simulink model "ADC_final_simulation"  (R2021a)
settings: Solver=ode4  StartTime=0.0  StopTime=50  FixedStep=0.01  RelTol=1e-3
libraries: mobileRoboticsLib x2, simulink x2, dspinverses x2, dsppolyfun x2
settings Model: Creator=rmml  LastModifiedBy=TigerWUU
settings SolverCC: ZeroCrossAlgorithm=Adaptive  AlgebraicLoopSolver=TrustRegion
settings DebuggingCC: IgnoredZcDiagnostic=none  SFMachineParentedDataDiag=warning

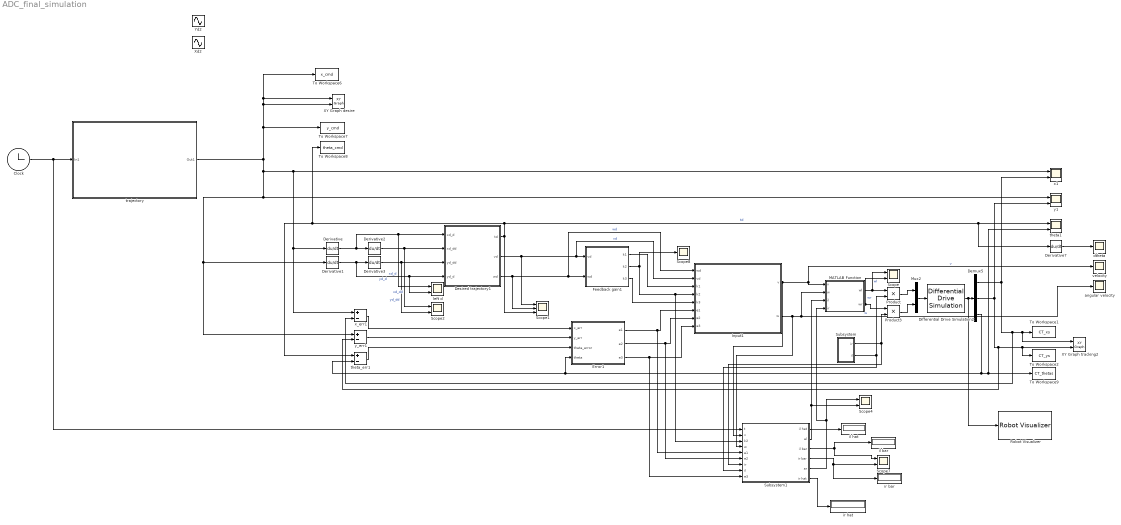
== system ADC_final_simulation ==
  Clock : Clock
  Demux5 : Demux  Outputs=3
  Derivative{,1..3,7} (5 alike) : Derivative  CoefficientInTFapproximation=0
  Desired trajectory1 : MATLAB Function  TreatAsAtomicUnit=on
  Differential Drive Simulation2 : mobileRoboticsLib/Kinematic Models/Differential Drive/Differential Drive Simulation  wheelRadius=0.075  wheelBase=0.3  initX=-0.2  initY=-0.2  initAngle=3*pi/4  Ts=0.01
      settings: SourceProductName=Mobile Robotics Simulation Toolbox
  Error1 : MATLAB Function  TreatAsAtomicUnit=on
  Feedback gain1 : MATLAB Function  TreatAsAtomicUnit=on
  Input1 : MATLAB Function  TreatAsAtomicUnit=on
  MATLAB Function : MATLAB Function  TreatAsAtomicUnit=on
  Mux2 : Mux  Inputs=2
  Product : Product
  Product3 : Product
  Robot Visualizer : mobileRoboticsLib/Environments/Robot Visualizer  robotRadius=0  showTrajectory=on  hasWaypoints=off  hasLidar=off  sensorOffset=[ 0, 0 ]  scanAngles=[ -pi/4, 0, pi/4 ]  hasObjDetector=off  objDetectorOffset=[ 0, 0 ]  objDetectorAngle=0  objDetectorFOV=pi/4  objDetectorMaxRange=5  objectColors=[ 1, 0, 0; 0, 1, 0; 0, 0, 1 ]  objectMarkers='s'
  Scope{,2,4,7} (4 alike) : Scope  NumInputPorts=2
  Scope1 : Scope  NumInputPorts=3
  Scope8 : Scope
  Subsystem : Subsystem
  Subsystem1 : Subsystem
  To Workspace1 : ToWorkspace  VariableName=CT_xs  SampleTime=-1
      settings: Save2DSignal=2-D array (concatenate along first dimension)
  To Workspace2 : ToWorkspace  VariableName=CT_ys  SampleTime=-1
      settings: Save2DSignal=2-D array (concatenate along first dimension)
  To Workspace6 : ToWorkspace  VariableName=x_cmd  SampleTime=-1
      settings: Save2DSignal=2-D array (concatenate along first dimension)
  To Workspace7 : ToWorkspace  VariableName=y_cmd  SampleTime=-1
      settings: Save2DSignal=2-D array (concatenate along first dimension)
  To Workspace8 : ToWorkspace  VariableName=theta_cmd  SampleTime=-1
      settings: Save2DSignal=2-D array (concatenate along first dimension)
  To Workspace9 : ToWorkspace  VariableName=CT_thetas  SampleTime=-1
      settings: Save2DSignal=2-D array (concatenate along first dimension)
  XY Graph desire : simulink/Sinks/XY Graph  xmin=-3  xmax=3  ymin=-3  ymax=3  st=-1
  XY Graph tracking2 : simulink/Sinks/XY Graph  xmin=-3  xmax=3  ymin=-3  ymax=3  st=-1
  Xd2 : Sin  TimeSource=Use external signal  Amplitude=-1.6  SampleTime=0
  Yd2 : Sin  TimeSource=Use external signal  Amplitude=-1.6  Bias=1.6  Phase=pi/2  SampleTime=0
  angular velocity : Scope
  dtheta : Scope
  il bar : Display
  il hat : Display
  ir bar : Display
  ir hat : Display
  left d : Scope  NumInputPorts=2
  theta1 : Scope  NumInputPorts=2
  theta_err1 : Sum  Inputs=+-
  trajectory : Subsystem
  velocity : Scope
  x1 : Scope  NumInputPorts=2
  x_err1 : Sum  Inputs=+-
  y1 : Scope  NumInputPorts=2
  y_err1 : Sum  Inputs=+-
  wires:
  Derivative/1 -> Derivative2/1, left d/1, Desired trajectory1/1(xd_d)  "xd_d"
  Derivative7/1 -> dtheta/1
  Feedback gain1/3(k3) -> Input1/5(k3)
  Derivative1/1 -> Desired trajectory1/4(yd_d), left d/2, Derivative3/1  "yd_d"
  Error1/1(e1) -> Subsystem1/5(e1), Input1/6(e1)
  Input1/1(v) -> Subsystem1/2(v), MATLAB Function/1(v), velocity/1  "v"
  y_err1/1 -> Error1/2(y_err)
  Error1/2(e2) -> Subsystem1/6(e2), Input1/7(e2)
  Desired trajectory1/1(td) -> To Workspace8/1, theta_err1/1, theta1/1, Derivative7/1, Scope1/3  "td"
  x_err1/1 -> Error1/1(x_err)
  Derivative2/1 -> Scope2/1, Desired trajectory1/2(xd_dd)  "xd_dd"
  Input1/2(w) -> Subsystem1/4(w), angular velocity/1, MATLAB Function/2(w)  "w"
  Desired trajectory1/2(vd) -> Scope1/1, Feedback gain1/1(vd), Input1/2(vd)  "vd"
  Feedback gain1/2(k2) -> Scope8/1, Subsystem1/3(k2), Input1/4(k2)
  Desired trajectory1/3(wd) -> Input1/1(wd), Feedback gain1/2(wd), Scope1/2  "wd"
  Clock/1 -> Subsystem1/1(t), trajectory/1(In1)
  Feedback gain1/1(k1) -> Input1/3(k1)
  Derivative3/1 -> Scope2/2, Desired trajectory1/3(yd_dd)  "yd_dd"
  Error1/3(e3) -> Subsystem1/9(e3), Input1/8(e3)
  theta_err1/1 -> Error1/3(theta_error)
  MATLAB Function/1(wl) -> Scope/1, Product/1  "wl"
  MATLAB Function/2(wr) -> Scope/2, Product3/1  "wr"
  Mux2/1 -> Differential Drive Simulation2/1
  Differential Drive Simulation2/1 -> Robot Visualizer/1, Demux5/1
  Demux5/1 -> x_err1/2, XY Graph tracking2/1, To Workspace1/1, x1/2
  Demux5/2 -> y_err1/2, To Workspace2/1, XY Graph tracking2/2, y1/2
  Product/1 -> Mux2/1
  Product3/1 -> Mux2/2
  Demux5/3 -> theta1/2, To Workspace9/1, Error1/4(theta), theta_err1/2
  trajectory/1(Out1) -> x1/1, x_err1/1, Derivative/1, Derivative1/1, y_err1/1, y1/1, To Workspace6/1, XY Graph desire/1, XY Graph desire/2, To Workspace7/1
  Subsystem/1(ir) -> Subsystem1/7(ir), Product3/2
  Subsystem/2(il) -> Subsystem1/8(il), Product/2
  Subsystem1/4(ir bar) -> ir bar/1, Scope7/2
  Subsystem1/3(il bar) -> Scope7/1, il bar/1
  Subsystem1/2(al) -> Scope4/2, MATLAB Function/3(il)
  Subsystem1/5(ar) -> MATLAB Function/4(ir), Scope4/1
  Subsystem1/1(il hat) -> il hat/1
  Subsystem1/6(ir hat) -> ir hat/1

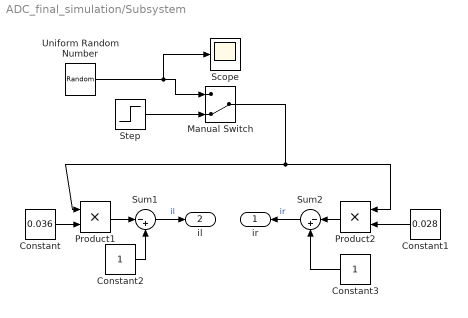
== system ADC_final_simulation/Subsystem ==
  Constant : Constant  Value=0.036
  Constant1 : Constant  Value=0.028
  Constant2 : Constant
  Constant3 : Constant
  Manual Switch : ManualSwitch  CurrentSetting=0
  Product1 : Product
  Product2 : Product
  Scope : Scope
  Step : Step  Time=20  SampleTime=0
  Sum1 : Sum  Inputs=|-+
  Sum2 : Sum  Inputs=|-+
  Uniform Random Number : UniformRandomNumber  SampleTime=0.1
  ir : Outport
  il : Outport  Port=2
  wires:
  Sum1/1 -> il/1  "il"
  Constant3/1 -> Sum2/2
  Product1/1 -> Sum1/1
  Product2/1 -> Sum2/1
  Constant2/1 -> Sum1/2
  Sum2/1 -> ir/1  "ir"
  Constant1/1 -> Product2/2
  Constant/1 -> Product1/2
  Step/1 -> Manual Switch/2
  Uniform Random Number/1 -> Scope/1, Manual Switch/1
  Manual Switch/1 -> Product2/1, Product1/1

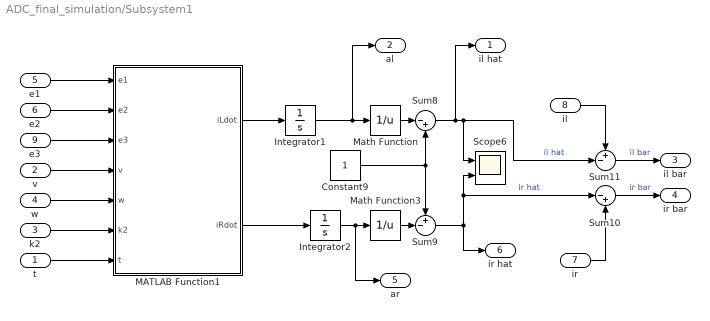
== system ADC_final_simulation/Subsystem1 ==
  t : Inport
  v : Inport  Port=2
  k2 : Inport  Port=3
  w : Inport  Port=4
  e1 : Inport  Port=5
  e2 : Inport  Port=6
  ir : Inport  Port=7
  il : Inport  Port=8
  e3 : Inport  Port=9
  Constant9 : Constant
  Integrator1 : Integrator
  Integrator2 : Integrator
  MATLAB Function1 : MATLAB Function  TreatAsAtomicUnit=on
  Math Function : Math  Operator=reciprocal  SaturateOnIntegerOverflow=on
  Math Function3 : Math  Operator=reciprocal  SaturateOnIntegerOverflow=on
  Scope6 : Scope  NumInputPorts=2
  Sum10 : Sum  Inputs=|-+
  Sum11 : Sum  Inputs=+-|
  Sum8 : Sum  Inputs=|-+
  Sum9 : Sum  Inputs=+-|
  il hat : Outport
  al : Outport  Port=2
  il bar : Outport  Port=3
  ir bar : Outport  Port=4
  ar : Outport  Port=5
  ir hat : Outport  Port=6
  wires:
  e2/1 -> MATLAB Function1/2(e2)
  Math Function/1 -> Sum8/1
  Integrator1/1 -> al/1, Math Function/1
  Integrator2/1 -> ar/1, Math Function3/1
  Constant9/1 -> Sum8/2, Sum9/1
  e3/1 -> MATLAB Function1/3(e3)
  w/1 -> MATLAB Function1/5(w)
  Sum8/1 -> il hat/1, Scope6/1, Sum11/2  "il hat"
  MATLAB Function1/2(iRdot) -> Integrator2/1
  Sum9/1 -> Scope6/2, Sum10/1, ir hat/1  "ir hat"
  Sum10/1 -> ir bar/1  "ir bar"
  t/1 -> MATLAB Function1/7(t)
  MATLAB Function1/1(iLdot) -> Integrator1/1
  Math Function3/1 -> Sum9/2
  Sum11/1 -> il bar/1  "il bar"
  k2/1 -> MATLAB Function1/6(k2)
  v/1 -> MATLAB Function1/4(v)
  e1/1 -> MATLAB Function1/1(e1)
  ir/1 -> Sum10/2
  il/1 -> Sum11/1

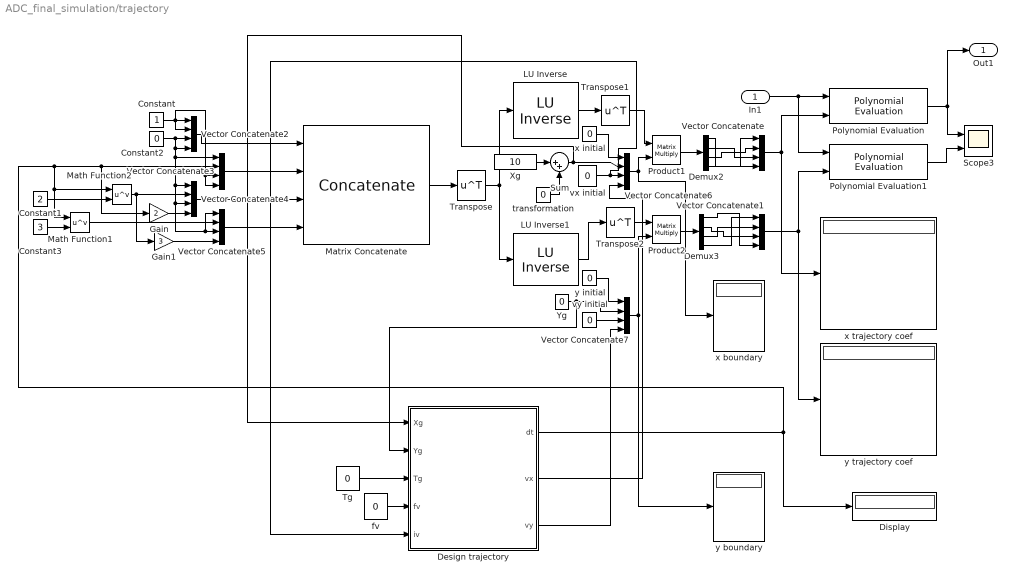
== system ADC_final_simulation/trajectory ==
  In1 : Inport
  " LU Inverse" : dspinverses/ LU Inverse
  " LU Inverse1" : dspinverses/ LU Inverse
  Constant : Constant
  Constant1 : Constant  Value=2
  Constant2 : Constant  Value=0
  Constant3 : Constant  Value=3
  Demux2 : Demux
  Demux3 : Demux
  Design trajectory : MATLAB Function  TreatAsAtomicUnit=on
  Display : Display
  Gain : Gain  Gain=2
  Gain1 : Gain  Gain=3
  Math Function1 : Math  Operator=pow  SaturateOnIntegerOverflow=on
  Math Function2 : Math  Operator=pow  SaturateOnIntegerOverflow=on
  Matrix Concatenate : Concatenate  NumInputs=4  Mode=Multidimensional array  ConcatenateDimension=2
  Polynomial Evaluation : dsppolyfun/Polynomial Evaluation  useConstCoeffs=off  constCoeffs=[5 4 3 2]
      settings: SourceProductBaseCode=DS
  Polynomial Evaluation1 : dsppolyfun/Polynomial Evaluation  useConstCoeffs=off  constCoeffs=[5 4 3 2]
      settings: SourceProductBaseCode=DS
  Product1 : Product  Multiplication=Matrix(*)
  Product2 : Product  Multiplication=Matrix(*)
  Scope3 : Scope  NumInputPorts=2
  Sum : Sum  Inputs=|++
  Tg : Constant  Value=0
  Transpose : Math  Operator=transpose  SaturateOnIntegerOverflow=on
  Transpose1 : Math  Operator=transpose  SaturateOnIntegerOverflow=on
  Transpose2 : Math  Operator=transpose  SaturateOnIntegerOverflow=on
  Vector Concatenate{,1..7} (8 alike) : Concatenate  NumInputs=4
  "Xg " : Constant  Value=10
  Yg : Constant  Value=0
  fv : Constant  Value=0
  transformation : Constant  Value=0
  "vx initial " : Constant  Value=0
  "vy initial " : Constant  Value=0
  "x boundary " : Display
  "x initial " : Constant  Value=0
  x trajectory coef : Display
  "y boundary " : Display
  "y initial " : Constant  Value=0
  y trajectory coef : Display
  Out1 : Outport
  wires:
  Polynomial Evaluation1/1 -> Scope3/2
  Product2/1 -> Demux3/1
  Yg/1 -> Design trajectory/2(Yg), Vector Concatenate7/2
  Math Function2/1 -> Gain1/1, Vector Concatenate4/2
  "vy initial "/1 -> Vector Concatenate7/3
  Tg/1 -> Design trajectory/3(Tg)
  Demux2/2 -> Vector Concatenate/3
  Constant/1 -> Vector Concatenate2/1, Vector Concatenate3/4, Vector Concatenate3/3, Vector Concatenate2/2
  fv/1 -> Design trajectory/4(fv)
  Vector Concatenate3/1 -> Matrix Concatenate/2
  Vector Concatenate5/1 -> Matrix Concatenate/4
  Vector Concatenate6/1 -> "x boundary "/1, Product1/2
  Vector Concatenate7/1 -> Product2/2, "y boundary "/1
  transformation/1 -> Sum/2
  Constant2/1 -> Vector Concatenate5/3, Vector Concatenate5/1, Vector Concatenate4/3, Vector Concatenate4/1, Vector Concatenate3/1, Vector Concatenate2/4, Vector Concatenate2/3
  Design trajectory/3(vy) -> Vector Concatenate7/4
  Transpose1/1 -> Product1/1
  "x initial "/1 -> Vector Concatenate6/1
  Demux3/4 -> Vector Concatenate1/1
  "Xg "/1 -> Sum/1
  " LU Inverse"/1 -> Transpose1/1
  " LU Inverse1"/1 -> Transpose2/1
  Product1/1 -> Demux2/1
  Vector Concatenate2/1 -> Matrix Concatenate/1
  "y initial "/1 -> Vector Concatenate7/1
  Demux2/3 -> Vector Concatenate/2
  Constant1/1 -> Math Function2/2
  Transpose2/1 -> Product2/1
  Matrix Concatenate/1 -> Transpose/1
  Vector Concatenate4/1 -> Matrix Concatenate/3
  Design trajectory/2(vx) -> Vector Concatenate6/4
  "vx initial "/1 -> Design trajectory/5(iv), Vector Concatenate6/3
  Polynomial Evaluation/1 -> Out1/1, Scope3/1
  Design trajectory/1(dt) -> Display/1, Math Function1/1, Math Function2/1, Vector Concatenate3/2, Gain/1
  Sum/1 -> Vector Concatenate6/2, Design trajectory/1(Xg)
  Transpose/1 -> " LU Inverse1"/1, " LU Inverse"/1
  In1/1 -> Polynomial Evaluation1/1, Polynomial Evaluation/1
  Constant3/1 -> Math Function1/2
  Math Function1/1 -> Vector Concatenate5/2
  Vector Concatenate1/1 -> y trajectory coef/1, Polynomial Evaluation1/2
  Gain/1 -> Vector Concatenate4/4
  Gain1/1 -> Vector Concatenate5/4
  Demux3/2 -> Vector Concatenate1/3
  Demux3/1 -> Vector Concatenate1/4
  Demux2/1 -> Vector Concatenate/4
  Demux3/3 -> Vector Concatenate1/2
  Vector Concatenate/1 -> x trajectory coef/1, Polynomial Evaluation/2
  Demux2/4 -> Vector Concatenate/1

== matlab function ADC_final_simulation/trajectory/Design trajectory ==
  data: Xg input; dt output; Yg input; Tg input; fv input; vx output; vy output; iv input
function [dt,vx,vy] = cmd_generation(Xg,Yg,Tg,fv,iv)

    distance = sqrt(Xg*Xg + Yg*Yg);
%     distance = 1.6*Xg;
    vx = sqrt((fv*fv)/(1+tan(Tg)*tan(Tg)));
    vy = vx*tan(Tg);
    dt = distance/0.05;
end

== matlab function ADC_final_simulation/MATLAB Function ==
  data: v input; wl output; w input; il input; ir input; wr output
function [wl,wr] = IK(v,w,il,ir)
    %parameters
    r=0.075;
    b=0.15;
    %inverse kinematics
%     wl = v/(r*il) - w*b/(r*il);
%     wr = v/(r*ir) + w*b/(r*ir);
    wl = v*il/(r) - w*b*il/(r);
    wr = v*ir/(r) + w*b*ir/(r);
end

== matlab function ADC_final_simulation/Subsystem1/MATLAB Function1 ==
  data: e1 input; iLdot output; e2 input; e3 input; v input; w input; iRdot output; k2 input; t input
function [iLdot,iRdot]  = observer(e1,e2,e3,v,w,k2,t)

    %parameters
    r=0.075;
    b=0.15;
    p1=20;
    p2=100;
    
    if (t<0.01)
    iLdot=0.1;
    iRdot=0.1;
    else
    iLdot=p1*((e2/b + 1/2)*e1*v - (e2/2 + b/4)*e1*w - sin(e3)/k2*(v/b - w/2));
    iRdot=p2*(-(e2/b - 1/2)*e1*v - (e2/2 - b/4)*e1*w + sin(e3)/k2*(v/b + w/2));

    end



end

== matlab function ADC_final_simulation/Desired trajectory1 ==
  data: xd_d input; td output; xd_dd input; yd_dd input; yd_d input; vd output; wd output
function [td,vd,wd] = cmd_generation(xd_d,xd_dd,yd_dd,yd_d)
%    if atan2(yd_d,xd_d)<0
%        td=atan2(yd_d,xd_d)+2*pi;
%    else
        td=atan2(yd_d,xd_d);
%    end
    vd = sqrt(xd_d^2+yd_d^2);
    if(xd_d^2+yd_d^2==0)
        wd=0;
    else
        wd=(yd_dd*xd_d-xd_dd*yd_d)/(xd_d^2+yd_d^2);
    end
end

== matlab function ADC_final_simulation/Error1 ==
  data: x_err input; e1 output; y_err input; theta_error input; theta input; e2 output; e3 output
function [e1,e2,e3] = error(x_err,y_err,theta_error,theta)
    e=[cos(theta) sin(theta) 0;-sin(theta) cos(theta) 0;0 0 1]*[x_err;y_err;theta_error];
    e1=e(1);
    e2=e(2);
    e3=e(3);
end

== matlab function ADC_final_simulation/Feedback gain1 ==
  data: k1 output; k2 output; k3 output; vd input; wd input
function [k1,k2,k3] = K(vd,wd)
    epsilon=1;
    b=14;
    
    k1=2*epsilon*sqrt(wd^2+b*vd^2);
    k3=k1;
    k2=b*abs(vd);
end

== matlab function ADC_final_simulation/Input1 ==
  data: wd input; vd input; v output; k1 input; k2 input; k3 input; e1 input; e2 input; e3 input; w output
function [v,w] = fcn(wd,vd,k1,k2,k3,e1,e2,e3)
    v=zeros(1);
    w=zeros(1);
    vmax=0.15;
    wmax=0.45;
    vc=vd*cos(e3)+k1*e1;
    wc=wd+k2*sign(vd)*e2+k3*e3;
%     wc=wd+k2*(vd)*e2+k3*sin(e3);

    sigma=max([abs(vc/vmax),abs(wc/wmax),1]);
    if(sigma==1)
        v=vc;
        w=wc;
    elseif(sigma==vc/vmax)
        v=sign(vc)*vmax;
        w=wc/sigma;
    else
        v=vc/sigma;
        w=sign(wc)*wmax;

    end
end
